simulink model "jednokompar"  (Simulink 8.0)
settings: Solver=ode45  StartTime=0.0  StopTime=40.0  RelTol=1e-3
settings Model: Creator=polacmi1  LastModifiedBy=Jarda
settings DataIOCC: SignalLoggingSaveFormat=ModelDataLogs
settings DebuggingCC: FcnCallInpInsideContextMsg=EnableAllAsWarning

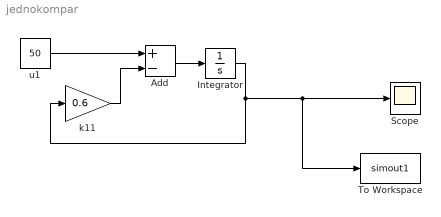
== system jednokompar ==
  Add : Sum  Inputs=+-
  Integrator : Integrator
  Scope : Scope
  To Workspace : ToWorkspace  VariableName=simout1  SampleTime=-1  SaveFormat=Timeseries
  k11 : Gain  Gain=0.6
  u1 : Constant  Value=50
  wires:
  k11/1 -> Add/2
  Integrator/1 -> k11/1, To Workspace/1, Scope/1
  Add/1 -> Integrator/1
  u1/1 -> Add/1
